simulink model "cmult_4bit_br_test"  (Simulink 7.0)
settings: Solver=VariableStepDiscrete  StartTime=0.0  StopTime=100  RelTol=1e-3
libraries: xbsIndex_r4 x11, casper_library x1
settings Model: Creator=User  LastModifiedBy=User
settings DebuggingCC: SaveWithDisabledLinksMsg=none  SaveWithParameterizedLinksMsg=none

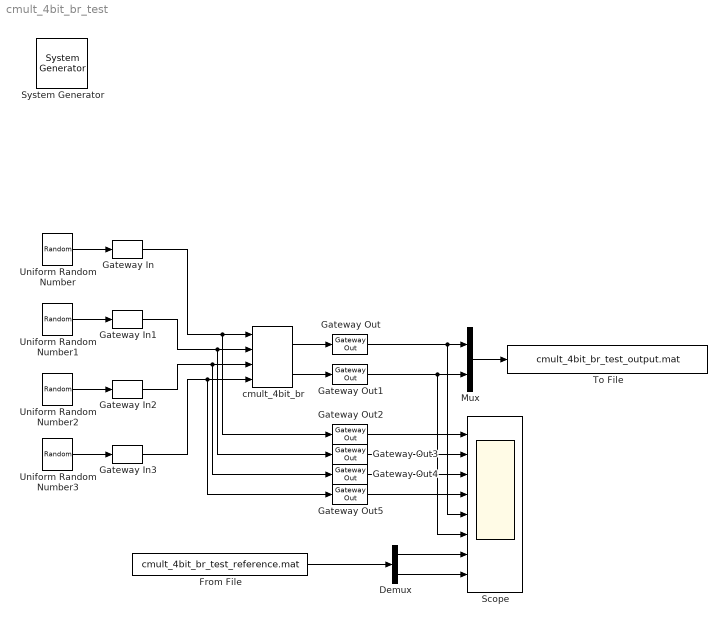
== system cmult_4bit_br_test ==
  " System Generator" : xbsIndex_r4/ System Generator  Tag=genX  SystemSampleTime=-1  xilinxfamily=Virtex4  part=xc4vsx35  speed=-10  package=ff668  synthesis_tool=XST  clock_wrapper=Clock Enables  directory=./netlist  testbench=off  simulink_period=1  sysclk_period=100  dcm_input_clock_period=100  incr_netlist=off  trim_vbits=Everywhere in SubSystem  dbl_ovrd=According to Block Masks  core_generation=According to Block Masks  run_coregen=off  deprecated_control=off  eval_field=0  block_type=sysgen
      settings: block_version=10.1.1
  Demux : Demux  Outputs=2
  From File : FromFile  FileName=cmult_4bit_br_test_reference.mat  SampleTime=1
  Gateway In{,1..3} (4 alike) : xbsIndex_r4/Gateway In  arith_type="Signed  (2's comp)"  n_bits=4  bin_pt=3  quantization=Truncate  overflow=Wrap  period=1  dbl_ovrd=off  timing_constraint=None  locs_specified=off  LOCs={}  block_type=gatewayin
      settings: infoedit="Gateway in block.  Converts inputs of type Simulink integer, double and fixed point to  Xilinx fixed point type.<P><P>Hardware notes:  In hardware these blocks become top level input ports."  block_version=10.1.1
  Gateway Out{,1..5} (6 alike) : xbsIndex_r4/Gateway Out  hdl_port=on  timing_constraint=None  locs_specified=off  LOCs={}  block_type=gatewayout
      settings: infoedit="Gateway out block.  Converts Xilinx fixed point inputs into ouputs of type Simulink integer, double, or fixed point.<P><P>Hardware notes:  In hardware these blocks become top level output ports or are discarded, depending on how they are configured."  block_version=10.1.1
  Mux : Mux  Inputs=2
  Scope : Scope  NumInputPorts=8
      settings: YMin=-1~-1~-1~-1~-2~-2~-2~-2  YMax=1~1~1~1~2~2~2~2
  To File : ToFile  Filename=cmult_4bit_br_test_output.mat  MatrixName=output
  Uniform Random Number : UniformRandomNumber  SampleTime=1
  Uniform Random Number1 : UniformRandomNumber  Seed=1  SampleTime=1
  Uniform Random Number2 : UniformRandomNumber  Seed=1  SampleTime=1
  Uniform Random Number3 : UniformRandomNumber  Seed=1  SampleTime=1
  cmult_4bit_br : casper_library/Multipliers/cmult_4bit_br  SystemSampleTime=-1  mult_latency=2  add_latency=2
  wires:
  Uniform Random Number/1 -> Gateway In/1
  Uniform Random Number1/1 -> Gateway In1/1
  Uniform Random Number2/1 -> Gateway In2/1
  Uniform Random Number3/1 -> Gateway In3/1
  Gateway In/1 -> Gateway Out2/1, cmult_4bit_br/1
  Gateway In1/1 -> Gateway Out3/1, cmult_4bit_br/2
  Gateway In2/1 -> Gateway Out4/1, cmult_4bit_br/3
  Gateway In3/1 -> Gateway Out5/1, cmult_4bit_br/4
  Gateway Out2/1 -> Scope/1
  Gateway Out3/1 -> Scope/2
  Gateway Out4/1 -> Scope/3
  Gateway Out5/1 -> Scope/4
  Gateway Out/1 -> Mux/1, Scope/5
  Gateway Out1/1 -> Mux/2, Scope/6
  Mux/1 -> To File/1
  Demux/1 -> Scope/7
  Demux/2 -> Scope/8
  cmult_4bit_br/1 -> Gateway Out/1
  cmult_4bit_br/2 -> Gateway Out1/1
  From File/1 -> Demux/1
